simulink model "Sistema_Tanque_JAM"  (R2024b)
settings: Solver=VariableStepAuto  StartTime=0.0  StopTime=100  RelTol=1e-3
libraries: simulink x1
settings Model: Creator=joleh  LastModifiedBy=joleh
settings DataIOCC: SaveOutput=off  SaveTime=off
settings RTWCC: RTWVerbose=off

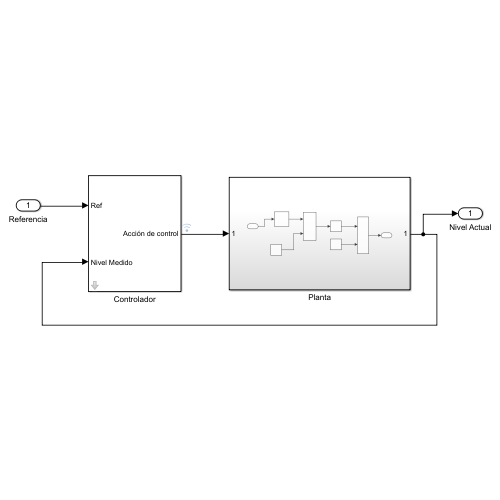
[thumbnail: Simulink's stored preview of the top-level diagram]
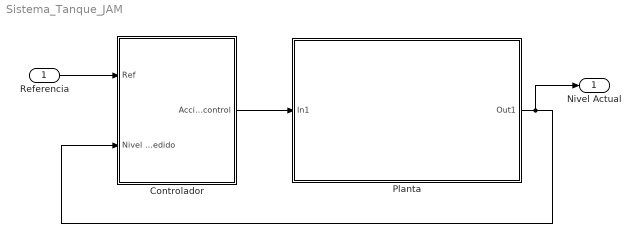
== system Sistema_Tanque_JAM ==
  Referencia : Inport  OutDataTypeStr=double  PortDimensions=1
  Controlador : Subsystem  mask{K_p=1}
  Planta : Subsystem
  Nivel Actual : Outport  OutDataTypeStr=double  PortDimensions=1  SampleTime=0
  wires:
  Controlador/1(Acción de control) -> Planta/1(In1)
  Planta/1(Out1) -> Controlador/2(Nivel Medido), Nivel Actual/1
  Referencia/1 -> Controlador/1(Ref)

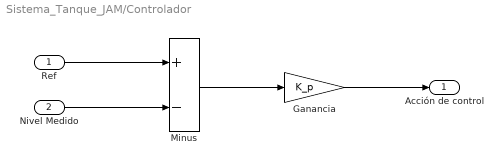
== system Sistema_Tanque_JAM/Controlador ==
  Ref : Inport
  Nivel Medido : Inport  Port=2
  Ganancia : Gain  Gain=K_p
  Minus : Sum  Inputs=+-
  Acción de control : Outport
  wires:
  Ganancia/1 -> Acción de control/1
  Nivel Medido/1 -> Minus/2
  Ref/1 -> Minus/1
  Minus/1 -> Ganancia/1

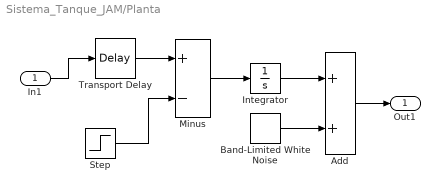
== system Sistema_Tanque_JAM/Planta ==
  In1 : Inport
  Add : Sum
  Band-Limited White Noise : simulink/Sources/Band-Limited White Noise  Cov=[0.1]  Ts=0.1  seed=[23341]
  Integrator : Integrator
  Minus : Sum  Inputs=+-
  Step : Step  After=0.1  SampleTime=0
  Transport Delay : TransportDelay
  Out1 : Outport
  wires:
  Add/1 -> Out1/1
  Integrator/1 -> Add/1
  Step/1 -> Minus/2
  Transport Delay/1 -> Minus/1
  In1/1 -> Transport Delay/1
  Minus/1 -> Integrator/1
  Band-Limited White Noise/1 -> Add/2
